simulink model "CLblock"  (R2016b)
settings: Solver=FixedStepAuto  StartTime=0.0  StopTime=simstop  MaxStep=0.1  RelTol=1e-3  EnableMultiTasking=on
undefined symbols (not defined in the file): CV01, input
libraries: xpcnilib x2, simulink x1
settings Model: ModifiedByFormat=The MathWorks Inc.  Creator=The MathWorks, Inc.  LastModifiedBy=The MathWorks Inc.
settings SolverCC: EnableConcurrentExecution=on
settings DataIOCC: LimitDataPoints=on  SaveFormat=Array
settings OptimizationCC: BlockReduction=off  DefaultParameterBehavior=Inlined  OptimizeBlockIOStorage=off  BufferReuse=off  GlobalBufferReuse=off  ExpressionFolding=off  ExpressionDepthLimit=2147483647  LocalBlockOutputs=off  LifeSpan=inf
settings DebuggingCC: UnderspecifiedInitializationDetection=Classic  MergeDetectMultiDrivingBlocksExec=none  SolverPrmCheckMsg=warning  FcnCallInpInsideContextMsg=warning  AllowSymbolicDim=off  StateNameClashWarn=warning  SFUnexpectedBacktrackingDiag=warning  SFNoUnconditionalDefaultTransitionDiag=warning  SFExecutionAtInitializationDiag=none
settings HardwareCC: ProdBitPerPointer=32  ProdBitPerSizeT=32  ProdBitPerPtrDiffT=32  ProdLargestAtomicFloat=None  ProdWordSize=32  ProdLongLongMode=on  ProdHWDeviceType=Generic->32-bit x86 compatible
settings ModelReferenceCC: ModelReferenceNumInstancesAllowed=Single  ModelReferenceMinAlgLoopOccurrences=on  PropagateSignalLabelsOutOfModel=off
settings RTWCC: SystemTargetFile=slrt.tlc  TemplateMakefile=slrt_default_tmf  Description=Simulink Real-Time  RTWVerbose=off
settings ConfigComp: CovMetricSettings=dw  CovHtmlReporting=on  CovSaveCumulativeToWorkspaceVar=on  CovSaveSingleToWorkspaceVar=on  CovExternalEMLEnable=off  CovSFcnEnable=off

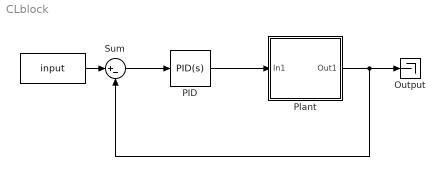
== system CLblock ==
  " " : Constant  Value=input
  Output : Terminator
  PID : simulink/Continuous/PID Controller  Controller=PID  TimeDomain=Continuous-time  SampleTime=-1  IntegratorMethod=Forward Euler  FilterMethod=Forward Euler  Form=Parallel  UseFilter=on  ControllerParametersSource=internal  P=1  I=1  D=0  N=100  InitialConditionSource=internal  InitialConditionForIntegrator=0  InitialConditionForFilter=0  ExternalReset=none  LimitOutput=off  UpperSaturationLimit=inf  LowerSaturationLimit=-inf  LinearizeAsGain=on  AntiWindupMode=none  Kb=1  TrackingMode=off  Kt=1  PParamMin=[]  PParamMax=[]  IParamMin=[]  IParamMax=[]  DParamMin=[]  DParamMax=[]  NParamMin=[]  NParamMax=[]  KbParamMin=[]  KbParamMax=[]  KtParamMin=[]  KtParamMax=[]  POutMin=[]  POutMax=[]  IOutMin=[]  IOutMax=[]  DOutMin=[]  DOutMax=[]  NOutMin=[]  NOutMax=[]  KbOutMin=[]  KbOutMax=[]  KtOutMin=[]  KtOutMax=[]  IntegratorOutMin=[]  IntegratorOutMax=[]  FilterOutMin=[]  FilterOutMax=[]  SumOutMin=[]  SumOutMax=[]  SumI1OutMin=[]  SumI1OutMax=[]  SumI2OutMin=[]  SumI2OutMax=[]  SumI3OutMin=[]  SumI3OutMax=[]  SumDOutMin=[]  SumDOutMax=[]  SaturationOutMin=[]  SaturationOutMax=[]  IntegratorContinuousStateAttributes=''  IntegratorStateMustResolveToSignalObject=off  IntegratorRTWStateStorageClass=Auto  FilterContinuousStateAttributes=''  FilterStateMustResolveToSignalObject=off  FilterRTWStateStorageClass=Auto  DifferentiatorICPrevScaledInput=0  DifferentiatorOutMin=[]  DifferentiatorOutMax=[]
  Plant : Subsystem
  Sum : Sum  Inputs=|+-
  wires:
  " "/1 -> Sum/1
  Sum/1 -> PID/1
  Plant/1(Out1) -> Output/1, Sum/2
  PID/1 -> Plant/1(In1)

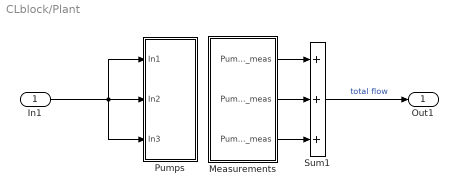
== system CLblock/Plant ==
  In1 : Inport
  Measurements : Subsystem
  Pumps : Subsystem
  Sum1 : Sum  Inputs=+++
  Out1 : Outport
  wires:
  Sum1/1 -> Out1/1  "total flow"
  In1/1 -> Pumps/3(In3), Pumps/2(In2), Pumps/1(In1)
  Measurements/1(Pump1_meas) -> Sum1/1
  Measurements/2(Pump2_meas) -> Sum1/2
  Measurements/3(Pump3_meas) -> Sum1/3

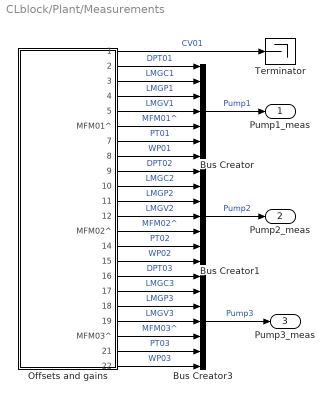
== system CLblock/Plant/Measurements ==
  Bus Creator : BusCreator  Inputs=7
  Bus Creator1 : BusCreator  Inputs=7
  Bus Creator3 : BusCreator  Inputs=7
  Offsets and gains : Subsystem
  Terminator : Terminator
  Pump1_meas : Outport
  Pump2_meas : Outport  Port=2
  Pump3_meas : Outport  Port=3
  wires:
  Bus Creator/1 -> Pump1_meas/1  "Pump1"
  Bus Creator1/1 -> Pump2_meas/1  "Pump2"
  Bus Creator3/1 -> Pump3_meas/1  "Pump3"
  Offsets and gains/8(8) -> Bus Creator/7  "WP01"
  Offsets and gains/9(9) -> Bus Creator1/1  "DPT02"
  Offsets and gains/4(4) -> Bus Creator/3  "LMGP1"
  Offsets and gains/2(2) -> Bus Creator/1  "DPT01"
  Offsets and gains/1(1) -> Terminator/1  "CV01"
  Offsets and gains/11(11) -> Bus Creator1/3  "LMGP2"
  Offsets and gains/15(15) -> Bus Creator1/7  "WP02"
  Offsets and gains/18(18) -> Bus Creator3/3  "LMGP3"
  Offsets and gains/22(22) -> Bus Creator3/7  "WP03"
  Offsets and gains/6(MFM01^) -> Bus Creator/5  "MFM01^"
  Offsets and gains/20(MFM03^) -> Bus Creator3/5  "MFM03^"
  Offsets and gains/10(10) -> Bus Creator1/2  "LMGC2"
  Offsets and gains/12(12) -> Bus Creator1/4  "LMGV2"
  Offsets and gains/13(MFM02^) -> Bus Creator1/5  "MFM02^"
  Offsets and gains/14(14) -> Bus Creator1/6  "PT02"
  Offsets and gains/19(19) -> Bus Creator3/4  "LMGV3"
  Offsets and gains/21(21) -> Bus Creator3/6  "PT03"
  Offsets and gains/16(16) -> Bus Creator3/1  "DPT03"
  Offsets and gains/17(17) -> Bus Creator3/2  "LMGC3"
  Offsets and gains/3(3) -> Bus Creator/2  "LMGC1"
  Offsets and gains/5(5) -> Bus Creator/4  "LMGV1"
  Offsets and gains/7(7) -> Bus Creator/6  "PT01"

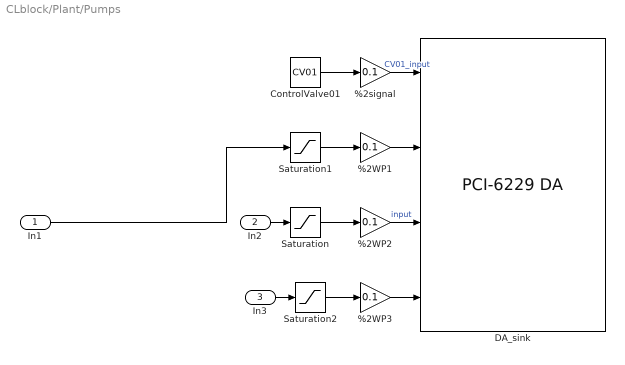
== system CLblock/Plant/Pumps ==
  In1 : Inport
  In2 : Inport  Port=2
  In3 : Inport  Port=3
  %2WP1 : Gain  Gain=0.1
  %2WP2 : Gain  Gain=0.1
  %2WP3 : Gain  Gain=0.1
  %2signal : Gain  Gain=0.1
  ControlValve01 : Constant  Value=CV01
  DA_sink : xpcnilib/D//A/M Series/PCI-6229 DA  channel=[4 1 2 3]  reset=[1]  initValue=[0]  sampletime=0.01  slot=-1
  Saturation : Saturate  UpperLimit=80  LowerLimit=0
  Saturation1 : Saturate  UpperLimit=80  LowerLimit=0
  Saturation2 : Saturate  UpperLimit=80  LowerLimit=0
  wires:
  In3/1 -> Saturation2/1
  In2/1 -> Saturation/1
  Saturation1/1 -> %2WP1/1
  Saturation2/1 -> %2WP3/1
  %2WP1/1 -> DA_sink/2
  %2WP3/1 -> DA_sink/4
  %2signal/1 -> DA_sink/1  "CV01_input"
  ControlValve01/1 -> %2signal/1
  %2WP2/1 -> DA_sink/3  "input"
  In1/1 -> Saturation1/1
  Saturation/1 -> %2WP2/1

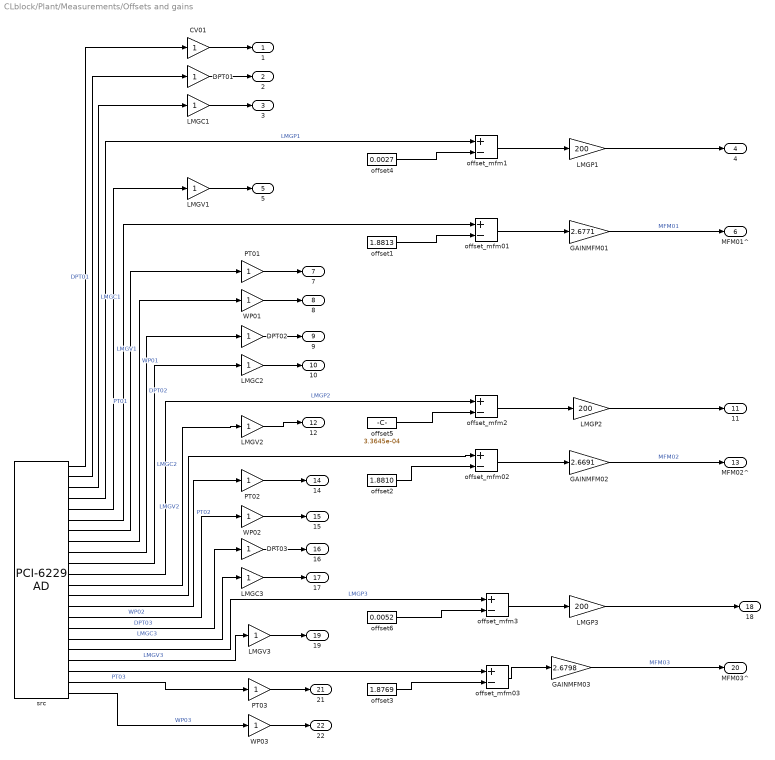
== system CLblock/Plant/Measurements/Offsets and gains ==
  CV01 : Gain
  DPT01 : Gain
  DPT02 : Gain
  DPT03 : Gain
  GAINMFM01 : Gain  Gain=2.6771
  GAINMFM02 : Gain  Gain=2.6691
  GAINMFM03 : Gain  Gain=2.6798
  LMGC1 : Gain
  LMGC2 : Gain
  LMGC3 : Gain
  LMGP1 : Gain  Gain=200
  LMGP2 : Gain  Gain=200
  LMGP3 : Gain  Gain=200
  LMGV1 : Gain
  LMGV2 : Gain
  LMGV3 : Gain
  PT01 : Gain
  PT02 : Gain
  PT03 : Gain
  WP01 : Gain
  WP02 : Gain
  WP03 : Gain
  offset1 : Constant  Value=1.8813
  offset2 : Constant  Value=1.8810
  offset3 : Constant  Value=1.8769
  offset4 : Constant  Value=0.0027
  offset5 : Constant  Value=3.3645e-04
  offset6 : Constant  Value=0.0052
  offset_mfm01 : Sum  Inputs=+-
  offset_mfm02 : Sum  Inputs=+-
  offset_mfm03 : Sum  Inputs=+-
  offset_mfm1 : Sum  Inputs=+-
  offset_mfm2 : Sum  Inputs=+-
  offset_mfm3 : Sum  Inputs=+-
  src : xpcnilib/A//D/M Series/PCI-6229 AD  channel=[4 17 5 11 8 21 24 1 18 6 12 9 22 25 2 19 7 13 10 23 26 3]  range=[10]  coupling=[0]  scantime=5e-6  sampletime=0.01  slot=-1
  1 : Outport
  2 : Outport  Port=2
  3 : Outport  Port=3
  4 : Outport  Port=4
  5 : Outport  Port=5
  MFM01^ : Outport  Port=6
  7 : Outport  Port=7
  8 : Outport  Port=8
  9 : Outport  Port=9
  10 : Outport  Port=10
  11 : Outport  Port=11
  12 : Outport  Port=12
  MFM02^ : Outport  Port=13
  14 : Outport  Port=14
  15 : Outport  Port=15
  16 : Outport  Port=16
  17 : Outport  Port=17
  18 : Outport  Port=18
  19 : Outport  Port=19
  MFM03^ : Outport  Port=20
  21 : Outport  Port=21
  22 : Outport  Port=22
  wires:
  src/18 -> offset_mfm3/1  "LMGP3"
  src/19 -> LMGV3/1  "LMGV3"
  src/22 -> WP03/1  "WP03"
  src/21 -> PT03/1  "PT03"
  src/10 -> LMGC2/1  "LMGC2"
  src/12 -> LMGV2/1  "LMGV2"
  src/15 -> WP02/1  "WP02"
  src/3 -> LMGC1/1  "LMGC1"
  src/9 -> DPT02/1  "DPT02"
  src/11 -> offset_mfm2/1  "LMGP2"
  src/14 -> PT02/1  "PT02"
  src/16 -> DPT03/1  "DPT03"
  src/17 -> LMGC3/1  "LMGC3"
  src/2 -> DPT01/1  "DPT01"
  src/1 -> CV01/1
  GAINMFM03/1 -> MFM03^/1  "MFM03"
  offset1/1 -> offset_mfm01/2
  src/4 -> offset_mfm1/1  "LMGP1"
  src/5 -> LMGV1/1  "LMGV1"
  src/7 -> PT01/1  "PT01"
  src/8 -> WP01/1  "WP01"
  offset3/1 -> offset_mfm03/2
  offset_mfm03/1 -> GAINMFM03/1
  offset_mfm01/1 -> GAINMFM01/1
  src/6 -> offset_mfm01/1
  src/20 -> offset_mfm03/1
  src/13 -> offset_mfm02/1
  offset_mfm02/1 -> GAINMFM02/1
  offset2/1 -> offset_mfm02/2
  GAINMFM02/1 -> MFM02^/1  "MFM02"
  GAINMFM01/1 -> MFM01^/1  "MFM01"
  CV01/1 -> 1/1
  DPT01/1 -> 2/1
  LMGC1/1 -> 3/1
  LMGV1/1 -> 5/1
  PT01/1 -> 7/1
  WP01/1 -> 8/1
  DPT02/1 -> 9/1
  LMGC2/1 -> 10/1
  LMGP2/1 -> 11/1
  LMGV2/1 -> 12/1
  PT02/1 -> 14/1
  WP02/1 -> 15/1
  DPT03/1 -> 16/1
  LMGC3/1 -> 17/1
  LMGP3/1 -> 18/1
  LMGV3/1 -> 19/1
  PT03/1 -> 21/1
  WP03/1 -> 22/1
  offset4/1 -> offset_mfm1/2
  offset_mfm1/1 -> LMGP1/1
  LMGP1/1 -> 4/1
  offset_mfm2/1 -> LMGP2/1
  offset5/1 -> offset_mfm2/2
  offset_mfm3/1 -> LMGP3/1
  offset6/1 -> offset_mfm3/2
